simulink model "Truckmodel"  (R2025b)
settings: Solver=VariableStepAuto  StartTime=0.0  StopTime=1  RelTol=1e-3
values from neighbouring files (symbols this model uses):
  b = 40e3    (= 40000)    [Simulink_assignment.m]
  k = 80.8e5    (= 8080000)    [Simulink_assignment.m]
  m = 0.033    [MATLAB_assignment.m]    (also in Simulink_assignment.m = 3000)
libraries: simulink x1
settings Model: Creator=zsong  LastModifiedBy=zsong

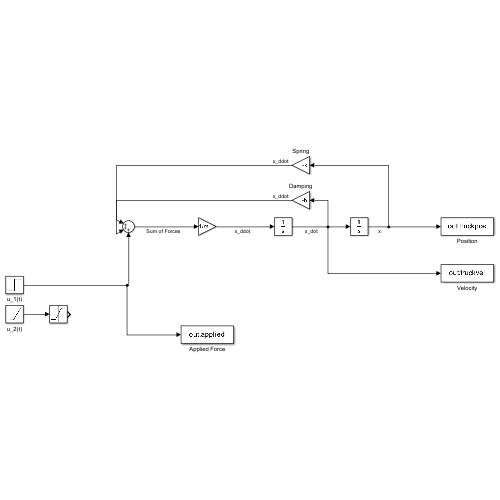
[thumbnail: Simulink's stored preview of the top-level diagram]
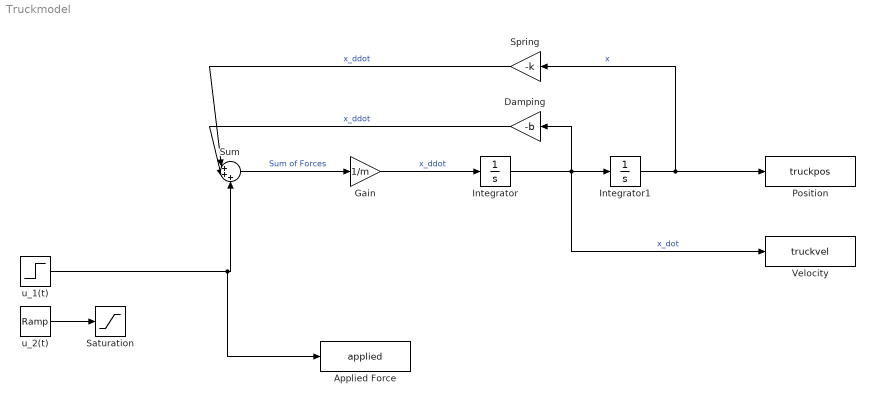
== system Truckmodel ==
  Applied Force : ToWorkspace  VariableName=applied  SampleTime=-1
  Damping : Gain  Gain=-b
  Gain : Gain  Gain=1/m
  Integrator : Integrator
  Integrator1 : Integrator
  Position : ToWorkspace  VariableName=truckpos  SampleTime=-1
  Saturation : Saturate  UpperLimit=u  LowerLimit=0
  Spring : Gain  Gain=-k
  Sum : Sum  Inputs=|+++
  Velocity : ToWorkspace  VariableName=truckvel  SampleTime=-1
  u_1(t) : Step  After=u  SampleTime=0
  u_2(t) : simulink/Sources/Ramp  slope=u  start=1  InitialOutput=0
  wires:
  Sum/1 -> Gain/1  "Sum of Forces"
  Gain/1 -> Integrator/1  "x_ddot"
  Integrator/1 -> Velocity/1, Integrator1/1, Damping/1  "x_dot"
  Integrator1/1 -> Position/1, Spring/1  "x"
  Spring/1 -> Sum/1  "x_ddot"
  Damping/1 -> Sum/2  "x_ddot"
  u_2(t)/1 -> Saturation/1
  u_1(t)/1 -> Applied Force/1, Sum/3
